simulink model "ExampleLights"  (Simulink 9.2)
settings: Solver=FixedStepDiscrete  StartTime=0.0  StopTime=inf  FixedStep=0.001  RelTol=1e-3  EnableMultiTasking=on
PostLoadFcn:
  | TIMESTEP = 0.001;
libraries: rFproPhysicsLib x7, simulink x4
settings Model: Creator=enewton  LastModifiedBy=SeanKavanagh
settings OptimizationCC: ExpressionDepthLimit=2147483647
settings DebuggingCC: SolverPrmCheckMsg=warning
settings RTWCC: SystemTargetFile=rfpro.tlc  MakeCommand="make_rtw OPTS=\"-DRUN_PHYSICS\""  TemplateMakefile=rfpro.tmf  Description=rFpro Target (Run Physics)  BuildConfiguration=Faster Runs  TargetLang=C++
settings STFCustomTargetCC: ModelReferenceCompliant=off  GeneratePreprocessorConditionals=Disable all  CombineOutputUpdateFcns=on  MatFileLogging=on  CPPClassGenCompliant=on  GRTInterface=off  SystemTargetFile=rfpro.tlc
settings GRTTargetCC: ModelReferenceCompliant=off  ParMdlRefBuildCompliant=off  CompOptLevelCompliant=off  ConcurrentExecutionCompliant=off  CombineOutputUpdateFcns=on  GRTInterface=off  UseToolchainInfoCompliant=off

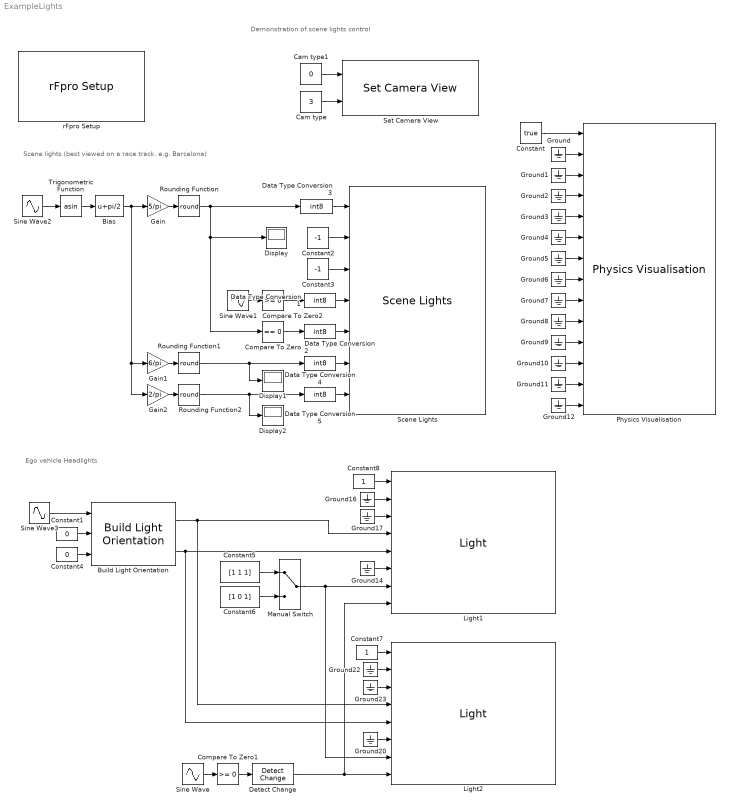
== system ExampleLights ==
  note: Demonstration of scene lights control
  note: Scene lights
      | (best viewed on a race track. e.g. Barcelona)
  note: Ego vehicle Headlights
  Bias : Bias  Bias=pi/2
  Build Light Orientation : rFproPhysicsLib/Build Light Orientation  isTypeC=off
  Cam type : Constant  Value=3
  Cam type1 : Constant  Value=0
  Compare To Zero : simulink/Logic and Bit Operations/Compare To Zero  relop===  OutDataTypeStr=boolean
  Compare To Zero1 : simulink/Logic and Bit Operations/Compare To Zero  relop=>=  OutDataTypeStr=uint8
  Compare To Zero2 : simulink/Logic and Bit Operations/Compare To Zero  relop=>=  OutDataTypeStr=uint8
  Constant : Constant  Value=true
  Constant1 : Constant  Value=0  OutDataTypeStr=double
  Constant2 : Constant  Value=-1  OutDataTypeStr=int8
  Constant3 : Constant  Value=-1  OutDataTypeStr=int8
  Constant4 : Constant  Value=0  OutDataTypeStr=double
  Constant5 : Constant  Value=[1 1 1]  OutDataTypeStr=double
  Constant6 : Constant  Value=[1 0 1]  OutDataTypeStr=double
  Constant7 : Constant
  Constant8 : Constant
  Data Type Conversion{1..5} (5 alike) : DataTypeConversion  OutDataTypeStr=int8
  Detect Change : simulink/Logic and Bit Operations/Detect Change  vinit=0  OutDataTypeStr=boolean
  Display : Display
  Display1 : Display
  Display2 : Display
  Gain : Gain  Gain=5/pi
  Gain1 : Gain  Gain=6/pi
  Gain2 : Gain  Gain=2/pi
  Ground{,1..12,14,16..17,20,22..23} (19 alike) : Ground
  Light1 : rFproPhysicsLib/Light  light_name='HighbeamL'  exact_match=on  on_vehicle=on  useReverseByteOrder=off  rFpro__platform=Remote Model - Default  posValid=off  dirValid=on  dirType=on  oriValid=on  intensityValid=off  colorValid=on
  Light2 : rFproPhysicsLib/Light  light_name='HighbeamR'  exact_match=on  on_vehicle=on  useReverseByteOrder=off  rFpro__platform=Remote Model - Default  posValid=off  dirValid=on  dirType=on  oriValid=on  intensityValid=off  colorValid=on
  Manual Switch : ManualSwitch
  Physics Visualisation : rFproPhysicsLib/Physics Visualisation  PAR_SKIP_INTERNAL_PHYSICS=off  PAR_ACCEL_VALID=off  PAR_ROT_ACCEL_VALID=off  PAR_GEAR_VALID=off  PAR_RPM_VALID=off  PAR_INPUTS_VALID=on  PAR_STEER_TORQUE_VALID=on  PAR_HEADLIGHTS_ON_VALID=off  PAR_WHEEL_POS_VALID=off  PAR_WHEEL_ORI_VALID=off  PAR_TYRE_PARAMS_VALID=off  PAR_WHEEL_ROTATION_VALID=off  PAR_WHEEL_BRAKE_TEMP_VALID=off  PAR_WHEEL_TREAD_TEMP_VALID=off  PAR_WHEEL_AIR_TEMP_VALID=off  period=-1  offset=0  useReverseByteOrder=on  rFpro__platform=Remote Model - Default
  Rounding Function : Rounding  Operator=round
  Rounding Function1 : Rounding  Operator=round
  Rounding Function2 : Rounding  Operator=round
  Scene Lights : rFproPhysicsLib/Scene Lights  packets_per_change=1  useReverseByteOrder=off  rFpro__platform=Remote Model - Default
  Set Camera View : rFproPhysicsLib/Set Camera View  triggerWidth=1  useReverseByteOrder=off  rFpro__platform=Remote Model - Default
  Sine Wave : Sin  Frequency=2*pi/0.01  SampleTime=0
  Sine Wave1 : Sin  Frequency=2*pi/2  SampleTime=0
  Sine Wave2 : Sin  Frequency=2*pi/5  Phase=pi/2  SampleTime=0
  Sine Wave3 : Sin  Amplitude=20  Frequency=2*pi  SampleTime=0
  Trigonometric Function : Trigonometry  Operator=asin
  rFpro Setup : rFproPhysicsLib/rFpro Setup  platform=Remote Model - Default  stopOnSessionEnd=on  usePseudoRealtime=on  syncToRF=on  useReverseByteOrder=off  useRfTime=on  minIterations=4  maxIterations=1000  ipReceiveAddress='127.0.0.1'  ipReceivePort=11054  receiveSampleTime=-1  ipTransmitAddress='127.0.0.1'  ipTransmitPort=11052  transmitSampleTime=-1  pluginType=RUN_PHYSICS  sysTarget=xpctarget.tlc  templateMakeFile=xpc_default_tmf  makeCommand=make_rtw  buildDesc=xPC target
  wires:
  Constant/1 -> Physics Visualisation/1
  Ground/1 -> Physics Visualisation/2
  Ground1/1 -> Physics Visualisation/3
  Ground2/1 -> Physics Visualisation/4
  Ground3/1 -> Physics Visualisation/5
  Ground4/1 -> Physics Visualisation/6
  Ground5/1 -> Physics Visualisation/7
  Ground6/1 -> Physics Visualisation/8
  Ground7/1 -> Physics Visualisation/9
  Ground8/1 -> Physics Visualisation/10
  Ground9/1 -> Physics Visualisation/11
  Ground10/1 -> Physics Visualisation/12
  Ground11/1 -> Physics Visualisation/13
  Constant2/1 -> Scene Lights/2
  Data Type Conversion3/1 -> Scene Lights/1
  Compare To Zero2/1 -> Data Type Conversion1/1
  Compare To Zero/1 -> Data Type Conversion2/1
  Rounding Function1/1 -> Display1/1, Data Type Conversion4/1
  Data Type Conversion1/1 -> Scene Lights/4
  Data Type Conversion4/1 -> Scene Lights/6
  Data Type Conversion2/1 -> Scene Lights/5
  Ground12/1 -> Physics Visualisation/14
  Rounding Function2/1 -> Display2/1, Data Type Conversion5/1
  Data Type Conversion5/1 -> Scene Lights/7
  Cam type/1 -> Set Camera View/2
  Cam type1/1 -> Set Camera View/1
  Constant3/1 -> Scene Lights/3
  Compare To Zero1/1 -> Detect Change/1
  Sine Wave/1 -> Compare To Zero1/1
  Sine Wave1/1 -> Compare To Zero2/1
  Trigonometric Function/1 -> Bias/1
  Bias/1 -> Gain2/1, Gain1/1, Gain/1
  Gain/1 -> Rounding Function/1
  Rounding Function/1 -> Data Type Conversion3/1, Display/1, Compare To Zero/1
  Gain1/1 -> Rounding Function1/1
  Gain2/1 -> Rounding Function2/1
  Ground17/1 -> Light1/3
  Manual Switch/1 -> Light1/7, Light2/7
  Ground14/1 -> Light1/6
  Ground16/1 -> Light1/2
  Ground23/1 -> Light2/3
  Ground20/1 -> Light2/6
  Ground22/1 -> Light2/2
  Sine Wave3/1 -> Build Light Orientation/1
  Constant1/1 -> Build Light Orientation/2
  Constant4/1 -> Build Light Orientation/3
  Constant5/1 -> Manual Switch/1
  Constant6/1 -> Manual Switch/2
  Build Light Orientation/2 -> Light1/5, Light2/5
  Build Light Orientation/1 -> Light1/4, Light2/4
  Detect Change/1 -> Light1/8, Light2/8
  Constant7/1 -> Light2/1
  Constant8/1 -> Light1/1
  Sine Wave2/1 -> Trigonometric Function/1
